simulink model "brush_proportionel"  (R2013a)
settings: Solver=ode45  StartTime=0.0  StopTime=2.0  RelTol=1e-3
libraries: powerlib x8, simulink x3, electricdrivelib x1
settings Model: Creator=hp  LastModifiedBy=hp

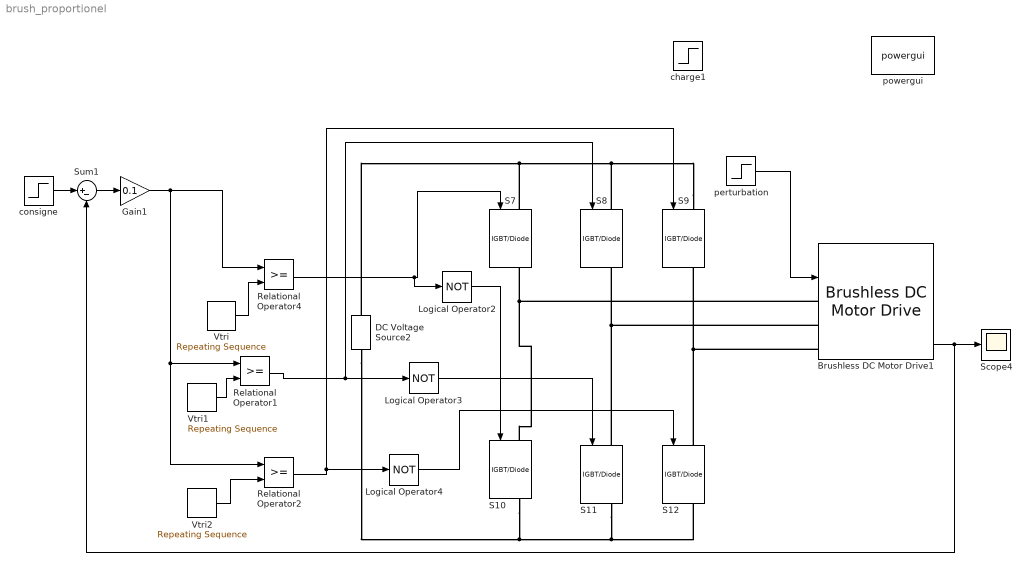
== system brush_proportionel ==
  Brushless DC Motor Drive1 : electricdrivelib/AC drives/Brushless DC Motor Drive  showMaskWarnings=on  AverageValue=off  MechanicalLoad=Torque Tm  driveType=AC7
  DC Voltage Source2 : powerlib/Electrical Sources/DC Voltage Source  Amplitude=240  Measurements=None
  Gain1 : Gain  Gain=0.1
  Logical Operator2 : Logic  Operator=NOT  AllPortsSameDT=off  OutDataTypeStr=boolean
  Logical Operator3 : Logic  Operator=NOT  AllPortsSameDT=off  OutDataTypeStr=boolean
  Logical Operator4 : Logic  Operator=NOT  AllPortsSameDT=off  OutDataTypeStr=boolean
  Relational Operator1 : RelationalOperator  OutDataTypeStr=boolean
  Relational Operator2 : RelationalOperator  OutDataTypeStr=boolean
  Relational Operator4 : RelationalOperator  OutDataTypeStr=boolean
  S{7..12} (6 alike) : powerlib/Power Electronics/IGBT//Diode  Ron=1e-3  Rs=1e5  Cs=inf  Measurements=on
  Scope4 : Scope
      settings: SaveName=vitesse
  Sum1 : Sum  Inputs=|+-
  Vtri : simulink/Sources/Repeating Sequence  rep_seq_t=[0 (1/2) 1]*0.001  rep_seq_y="[-1  1 -1] *240"
  Vtri1 : simulink/Sources/Repeating Sequence  rep_seq_t=[0 (1/6) 1]*0.001  rep_seq_y="[-1  1 -1] *240"
  Vtri2 : simulink/Sources/Repeating Sequence  rep_seq_t=[0 (1/3) 1]*0.001  rep_seq_y="[-1  1 -1] *240"
  charge1 : Step  Time=0.1  After=0.1  SampleTime=0
  consigne : Step  Time=0  After=150  SampleTime=0
  perturbation : Step  Time=0.2  After=10  SampleTime=0
  powergui : powerlib/powergui  Priority=1  SimulationMode=Discrete  SolverType=Tustin  SampleTime=1e-6  frequency=60  SPID=off  DisableSnubberDevices=off  DisableRonSwitches=off  DisableVfSwitches=off  SwTol=0  Interpol=off  DisplayEquations=off  frequencyindice=0  Pbase=100e6  ErrMax=1e-4  Iterations=50  UnitsV=kV  UnitsW=MW  FunctionMessages=off  echomessages=off  HookPort=off  EnableUseOfTLC=off  x0status=blocks  RestoreLinks=warning  ResistiveCurrentMeasurement=off  Frange=[0:2:500]  Ylog=off  Xlog=on  ShowGrid=off  save=off  variable=ZData  ZoomFFT=off  StartTime=0.0  cycles=1  DisplayStyle=1  fundamental=60  FreqAxis=off  MaxFrequency=1000  frequencyindicesteady=1  RmsSteady=1  display=off  Ts=0  methode=off
  wires:
  Relational Operator4/1 -> Logical Operator2/1, S7/1
  Logical Operator2/1 -> S10/1
  Relational Operator1/1 -> S8/1, Logical Operator3/1
  Logical Operator3/1 -> S11/1
  Relational Operator2/1 -> Logical Operator4/1, S9/1
  Logical Operator4/1 -> S12/1
  Vtri1/1 -> Relational Operator1/2
  Gain1/1 -> Relational Operator2/1, Relational Operator1/1, Relational Operator4/1
  Vtri2/1 -> Relational Operator2/2
  Vtri/1 -> Relational Operator4/2
  consigne/1 -> Sum1/1
  Sum1/1 -> Gain1/1
  Brushless DC Motor Drive1/4 -> Sum1/2, Scope4/1
  perturbation/1 -> Brushless DC Motor Drive1/2
  connections:
  S9/RConn1 -- S12/LConn1 -- Brushless DC Motor Drive1/LConn3
  S12/RConn1 -- S11/RConn1 -- DC Voltage Source2/LConn1 -- S10/RConn1
  S9/LConn1 -- S8/LConn1 -- DC Voltage Source2/RConn1 -- S7/LConn1
  S7/RConn1 -- S10/LConn1 -- Brushless DC Motor Drive1/LConn1
  S8/RConn1 -- S11/LConn1 -- Brushless DC Motor Drive1/LConn2
